simulink model "Project_Model_simulink_version_7_7_2023"  (R2021a)
settings: Solver=FixedStepDiscrete  StartTime=0.0  StopTime=10  FixedStep=0.2  RelTol=1e-3
undefined symbols (not defined in the file or in its folder): sigbuilder_block
(part 1 of 2)
settings Model: Creator=A  LastModifiedBy=91855
settings SolverCC: AlgebraicLoopSolver=TrustRegion

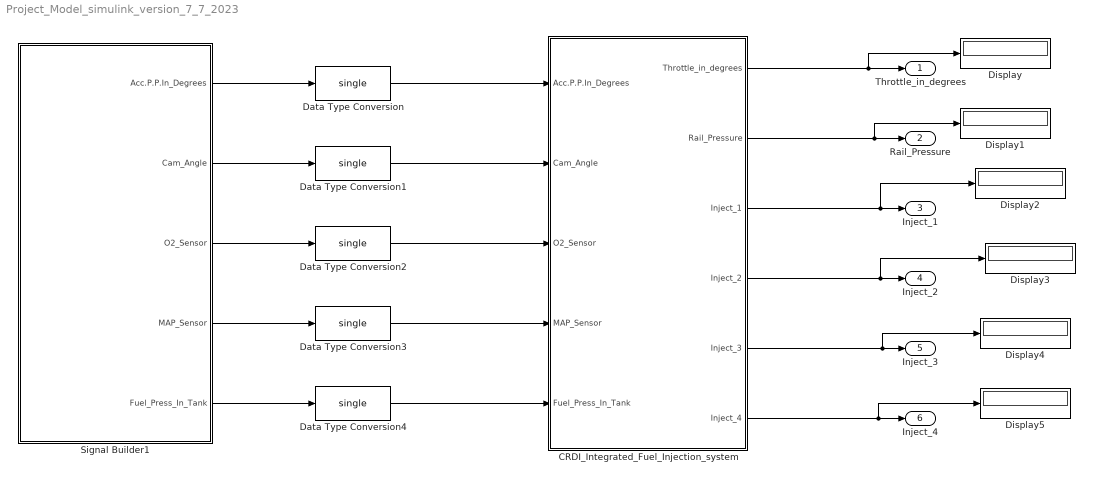
== system Project_Model_simulink_version_7_7_2023 ==
  CRDI_Integrated_Fuel_Injection_system : Subsystem
  Data Type Conversion{,1..4} (5 alike) : DataTypeConversion  OutDataTypeStr=single
  Display{,1..5} (6 alike) : Display
  Signal Builder1 : Subsystem  Tag=STV Subsys  LoadFcn=sigbuilder_block('load');  StartFcn=sigbuilder_block('start');  StopFcn=sigbuilder_block('stop');  ClipboardFcn=sigbuilder_block('clipboard');  mask(Sigbuilder block){tuvar=[0:10]}
      mask help: Simulink:masks:SigbuilderBlock_MD
      mask init:
      | if ~strcmp(get_param(bdroot(gcbh),'SimulationStatus'),'stopped') tuvar = sigbuilder_block('maskInit'); end
      settings: CopyFcn=sigbuilder_block('copy');  DeleteFcn=sigbuilder_block('delete');  ModelCloseFcn=sigbuilder_block('modelClose');  PreSaveFcn=sigbuilder_block('preSave');  PauseFcn=sigbuilder_block('pause');  ContinueFcn=sigbuilder_block('continue');  NameChangeFcn=sigbuilder_block('namechange');  OpenFcn=sigbuilder_block('open',[215 94 550.5 362.5 ]);  CloseFcn=sigbuilder_block('close');
      mask Display: plot(0, 0, 100, 100,[2, 2, 32, 32, 2], [68, 8, 8, 68, 68],[32, 2], [38, 38], [32, 19, 2],[53, 60, 44], [32, 17, 17, 2],[16, 16, 31, 31]);txt = getActiveGroup(gcbh);text(2, 100, txt,'verticalAlignment', 'top');
  Throttle_in_degrees : Outport  OutDataTypeStr=single
  Rail_Pressure : Outport  Port=2  OutDataTypeStr=single
  Inject_1 : Outport  Port=3  OutDataTypeStr=single
  Inject_2 : Outport  Port=4  OutDataTypeStr=single
  Inject_3 : Outport  Port=5  OutDataTypeStr=single
  Inject_4 : Outport  Port=6  OutDataTypeStr=single
  wires:
  CRDI_Integrated_Fuel_Injection_system/1(Throttle_in_degrees) -> Display/1, Throttle_in_degrees/1
  CRDI_Integrated_Fuel_Injection_system/2(Rail_Pressure) -> Display1/1, Rail_Pressure/1
  CRDI_Integrated_Fuel_Injection_system/3(Inject_1) -> Display2/1, Inject_1/1
  CRDI_Integrated_Fuel_Injection_system/4(Inject_2) -> Display3/1, Inject_2/1
  CRDI_Integrated_Fuel_Injection_system/5(Inject_3) -> Display4/1, Inject_3/1
  CRDI_Integrated_Fuel_Injection_system/6(Inject_4) -> Display5/1, Inject_4/1
  Data Type Conversion/1 -> CRDI_Integrated_Fuel_Injection_system/1(Acc.P.P.In_Degrees)
  Signal Builder1/2(Cam_Angle) -> Data Type Conversion1/1
  Signal Builder1/3(O2_Sensor) -> Data Type Conversion2/1
  Signal Builder1/4(MAP_Sensor) -> Data Type Conversion3/1
  Signal Builder1/5(Fuel_Press_In_Tank) -> Data Type Conversion4/1
  Data Type Conversion1/1 -> CRDI_Integrated_Fuel_Injection_system/2(Cam_Angle)
  Data Type Conversion2/1 -> CRDI_Integrated_Fuel_Injection_system/3(O2_Sensor)
  Data Type Conversion3/1 -> CRDI_Integrated_Fuel_Injection_system/4(MAP_Sensor)
  Data Type Conversion4/1 -> CRDI_Integrated_Fuel_Injection_system/5(Fuel_Press_In_Tank)
  Signal Builder1/1(Acc.P.P.In_Degrees) -> Data Type Conversion/1

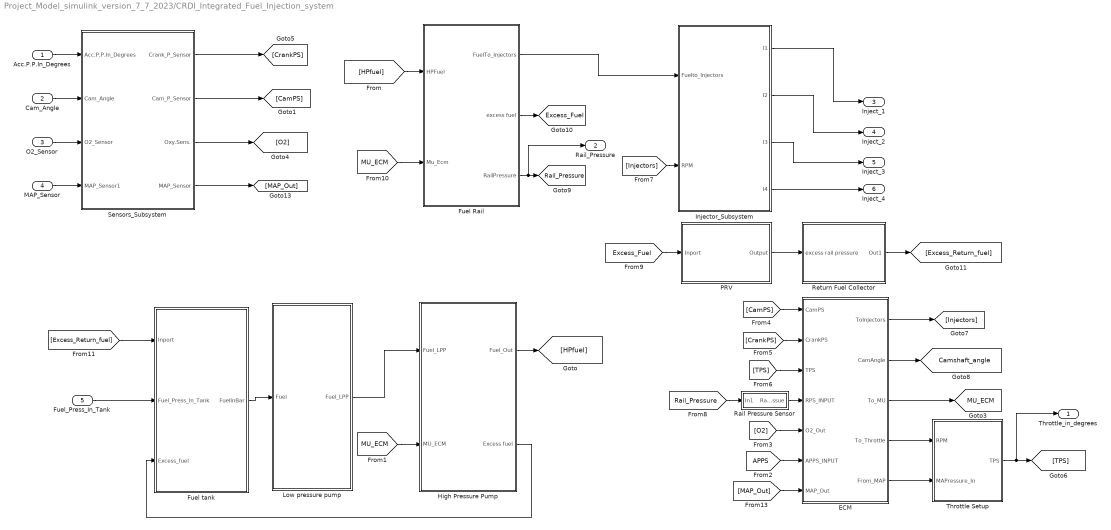
== system Project_Model_simulink_version_7_7_2023/CRDI_Integrated_Fuel_Injection_system ==
  Acc.P.P.In_Degrees : Inport  OutDataTypeStr=single
  Cam_Angle : Inport  Port=2  OutDataTypeStr=single
  O2_Sensor : Inport  Port=3  OutDataTypeStr=single
  MAP_Sensor : Inport  Port=4  OutDataTypeStr=single
  Fuel_Press_In_Tank : Inport  Port=5  OutDataTypeStr=single
  ECM : Subsystem
  Fuel Rail : Subsystem
  Fuel tank : Subsystem
  High Pressure Pump : Subsystem
  Injector_Subsystem : Subsystem
  Low pressure pump : Subsystem
  PRV : Subsystem
  Rail Pressure Sensor : Subsystem
  Return Fuel Collector : Subsystem
  Sensors_Subsystem : Subsystem
  Throttle Setup : Subsystem
  Throttle_in_degrees : Outport
  Rail_Pressure : Outport  Port=2
  Inject_1 : Outport  Port=3
  Inject_2 : Outport  Port=4
  Inject_3 : Outport  Port=5
  Inject_4 : Outport  Port=6
  tag scope: Camshaft_angle=global, Excess_Fuel=global, MU_ECM=global, Rail_Pressure=global
  wires:
  [MAP_Out] -> ECM/7(MAP_Out)
  [HPfuel] -> Fuel Rail/1(HPFuel)
  [Excess_Fuel] -> PRV/1(Inport)
  [Injectors] -> Injector_Subsystem/2(RPM)
  Throttle Setup/1(TPS) -> Throttle_in_degrees/1, [TPS]
  [O2] -> ECM/5(O2_Out)
  [MU_ECM] -> High Pressure Pump/2(MU_ECM)
  [Excess_Return_fuel] -> Fuel tank/1(Inport)
  [CamPS] -> ECM/1(CamPS)
  Rail Pressure Sensor/1(Rail Pressue) -> ECM/4(RPS_INPUT)
  [TPS] -> ECM/3(TPS)
  Fuel Rail/1(FuelTo_Injectors) -> Injector_Subsystem/1(Fuelto_Injectors)
  High Pressure Pump/2(Excess fuel) -> Fuel tank/3(Excess_fuel)
  [CrankPS] -> ECM/2(CrankPS)
  Fuel tank/1(FuelInBar) -> Low pressure pump/1(Fuel)
  Low pressure pump/1(Fuel_LPP) -> High Pressure Pump/1(Fuel_LPP)
  ECM/4(To_Throttle) -> Throttle Setup/1(RPM)
  ECM/1(ToInjectors) -> [Injectors]
  Return Fuel Collector/1(Out1) -> [Excess_Return_fuel]
  ECM/2(CamAngle) -> [Camshaft_angle]
  Fuel Rail/3(RailPressure) -> Rail_Pressure/1, [Rail_Pressure]
  High Pressure Pump/1(Fuel_Out) -> [HPfuel]
  ECM/3(To_MU) -> [MU_ECM]
  [Rail_Pressure] -> Rail Pressure Sensor/1(In1)
  Sensors_Subsystem/3(Oxy.Sens.) -> [O2]
  Sensors_Subsystem/2(Cam_P_Sensor) -> [CamPS]
  Fuel Rail/2(excess fuel) -> [Excess_Fuel]
  ECM/5(From_MAP) -> Throttle Setup/2(MAPressure_In)
  [APPS] -> ECM/6(APPS_INPUT)
  Sensors_Subsystem/1(Crank_P_Sensor) -> [CrankPS]
  Sensors_Subsystem/4(MAP_Sensor) -> [MAP_Out]
  PRV/1(Output) -> Return Fuel Collector/1(excess rail pressure)
  Injector_Subsystem/1(I1) -> Inject_1/1
  Injector_Subsystem/2(I2) -> Inject_2/1
  Injector_Subsystem/3(I3) -> Inject_3/1
  Injector_Subsystem/4(I4) -> Inject_4/1
  Fuel_Press_In_Tank/1 -> Fuel tank/2(Fuel_Press_In_Tank)
  O2_Sensor/1 -> Sensors_Subsystem/3(O2_Sensor)
  Cam_Angle/1 -> Sensors_Subsystem/2(Cam_Angle)
  MAP_Sensor/1 -> Sensors_Subsystem/4(MAP_Sensor1)
  Acc.P.P.In_Degrees/1 -> Sensors_Subsystem/1(Acc.P.P.In_Degrees)
  [MU_ECM] -> Fuel Rail/2(Mu_Ecm)

== system Project_Model_simulink_version_7_7_2023/Signal Builder1 ==
  Demux : Demux  Tag=STV Demux  Outputs=5
      settings: DisplayOption=none
  FromWs : FromWorkspace  Tag=STV FromWs  VariableName=tuvar
      SigBuilderData=|
      | common.afterFinalStr = 'Extrapolate'
      | common.sampleTime = 0
      | dataSet.timeRange = [0 4]
      | dataSet.name = 'Sheet2'
      | sbobj.Groups.Name = 'Sheet2'
      | sbobj.Groups.Signals(1).Name = 'Acc.P.P.In_Degrees'
      | sbobj.Groups.Signals(1).XData = [0 0.2 0.4 0.6 0.8 1 1.2 1.4 1.6 1.8 2 2.2 2.4 2.6 2.8 3 3.2 3.4 3.6 3.8 4]
      | sbobj.Groups.Signals(1).YData = [0 10 12 14 16 18 20 22 24 26 28 30 52 56 60 66 70 78 82 86 90]
      | sbobj.Groups.Signals(2).Name = 'Cam_Angle'
      | sbobj.Groups.Signals(2).XData = [0 0.2 0.4 0.6 0.8 1 1.2 1.4 1.6 1.8 2 2.2 2.4 2.6 2.8 3 3.2 3.4 3.6 3.8 4]
      | sbobj.Groups.Signals(2).YData = [177.5 179 180 183 184.5 222 224 225 229 267 269 270 272 274.5 313 314 315 319.2 340 345 350]
      | sbobj.Groups.Signals(3).Name = 'O2_Sensor'
      | sbobj.Groups.Signals(3).XData = [0 0.2 0.4 0.6 0.8 1 1.2 1.4 1.6 1.8 2 2.2 2.4 2.6 2.8 3 3.2 3.4 3.6 3.8 4]
      | sbobj.Groups.Signals(3).YData = [0.6 0.65 0.85 0.45 0.46 0.65 0.34 0.36 0.55 0.65 0.64 0.67 0.78 0.54 0.44 0.6 0.73 0.3 0.25 0.2 0.26]
      | sbobj.Groups.Signals(4).Name = 'MAP_Sensor'
      | sbobj.Groups.Signals(4).XData = [0 0.2 0.4 0.6 0.8 1 1.2 1.4 1.6 1.8 2 2.2 2.4 2.6 2.8 3 3.2 3.4 3.6 3.8 4]
      | sbobj.Groups.Signals(4).YData = [24 24.15 24.3 24.45 24.5 24.75 24.9 25.05 25.2 25.35 25.5 25.5 27.3 27.6 27.9 28.1 28.65 29.25 29.55 29.85 30]
      | sbobj.Groups.Signals(5).Name = 'Fuel_Press_In_Tank'
      | sbobj.Groups.Signals(5).XData = [0 0.2 0.4 0.6 0.8 1 1.2 1.4 1.6 1.8 2 2.2 2.4 2.6 2.8 3 3.2 3.4 3.6 3.8 4]
      | sbobj.Groups.Signals(5).YData = [1 1 1 1 1 1 1 1 1 1 1 1 1 1 1 1 1 1 1 1 1]
  Acc.P.P.In_Degrees : Outport  Tag=STV Outport
  Cam_Angle : Outport  Tag=STV Outport  Port=2
  O2_Sensor : Outport  Tag=STV Outport  Port=3
  MAP_Sensor : Outport  Tag=STV Outport  Port=4
  Fuel_Press_In_Tank : Outport  Tag=STV Outport  Port=5
  wires:
  Demux/1 -> Acc.P.P.In_Degrees/1
  FromWs/1 -> Demux/1
  Demux/2 -> Cam_Angle/1
  Demux/3 -> O2_Sensor/1
  Demux/4 -> MAP_Sensor/1
  Demux/5 -> Fuel_Press_In_Tank/1

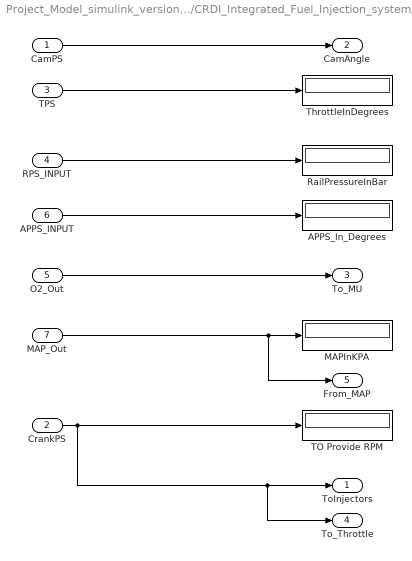
== system Project_Model_simulink_version_7_7_2023/CRDI_Integrated_Fuel_Injection_system/ECM ==
  CamPS : Inport  OutDataTypeStr=single
  CrankPS : Inport  Port=2
  TPS : Inport  Port=3
  RPS_INPUT : Inport  Port=4
  O2_Out : Inport  Port=5
  APPS_INPUT : Inport  Port=6
  MAP_Out : Inport  Port=7
  APPS_In_Degrees : Display
  MAPInKPA : Display
  RailPressureInBar : Display
  TO Provide RPM : Display
  ThrottleInDegrees : Display
  ToInjectors : Outport
  CamAngle : Outport  Port=2
  To_MU : Outport  Port=3
  To_Throttle : Outport  Port=4
  From_MAP : Outport  Port=5
  wires:
  CamPS/1 -> CamAngle/1
  APPS_INPUT/1 -> APPS_In_Degrees/1
  MAP_Out/1 -> From_MAP/1, MAPInKPA/1
  TPS/1 -> ThrottleInDegrees/1
  RPS_INPUT/1 -> RailPressureInBar/1
  CrankPS/1 -> To_Throttle/1, ToInjectors/1, TO Provide RPM/1
  O2_Out/1 -> To_MU/1

== system Project_Model_simulink_version_7_7_2023/CRDI_Integrated_Fuel_Injection_system/Fuel Rail ==
  HPFuel : Inport
  Mu_Ecm : Inport  Port=2
  1-D Lookup Table : Lookup_n-D  NumberOfTableDimensions=1  BreakpointsForDimension1=|  Table=|  InternalRulePriority=Speed  RndMeth=Simplest  InputSameDT=on
      BreakpointsForDimension1=|
      | [600
      | 730
      | 860
      | 990
      | 1120
      | 1250
      | 1380
      | 1510
      | 1640
      | 1770
      | 1900
      | 2030
      | 2160
      | 2290
      | 2420
      | 2550
      | 2680
      | 2810
      | 2940
      | 3070
      | 3200
      | 3330
      | 3460
      | 3590
      | 3720
      | 3850
      | 3980
      | 4110
      | 4240
      | 4370
      | 4500
      | 4630
      | 4760
      | 4890
      | 5020
      | 5150
      | 5280
      | 5410
      | 5540
      | 5670
      | 5800
      | 6000]
      Table=|
      | [300
      | 332
      | 364
      | 396
      | 428
      | 460
      | 492
      | 524
      | 556
      | 588
      | 620
      | 652
      | 684
      | 716
      | 748
      | 780
      | 812
      | 844
      | 876
      | 908
      | 940
      | 972
      | 1004
      | 1036
      | 1068
      | 1100
      | 1132
      | 1164
      | 1196
      | 1228
      | 1260
      | 1292
      | 1324
      | 1356
      | 1388
      | 1420
      | 1452
      | 1484
      | 1516
      | 1548
      | 1580
      | 1600]
  Product : Product
  Product1 : Product
  Subtract : Sum  Inputs=-+
  Subtract1 : Sum  Inputs=-+
  FuelTo_Injectors : Outport
  excess fuel : Outport  Port=2
  RailPressure : Outport  Port=3
  wires:
  1-D Lookup Table/1 -> Product/1, Subtract/1
  [RPM] -> 1-D Lookup Table/1
  HPFuel/1 -> Subtract1/2, Subtract/2
  Subtract/1 -> Subtract1/1, excess fuel/1
  Subtract1/1 -> Product1/1
  Product/1 -> RailPressure/1
  Product1/1 -> FuelTo_Injectors/1
  Mu_Ecm/1 -> Product1/2, Product/2

== system Project_Model_simulink_version_7_7_2023/CRDI_Integrated_Fuel_Injection_system/Fuel tank ==
  Inport : Inport
  Fuel_Press_In_Tank : Inport  Port=2
  Excess_fuel : Inport  Port=3
  ExcessFuelInBar : Display
  ExcessFuelInBar1 : Display
  FuelInBar : Outport
  wires:
  Inport/1 -> ExcessFuelInBar1/1
  Excess_fuel/1 -> ExcessFuelInBar/1
  Fuel_Press_In_Tank/1 -> FuelInBar/1

== system Project_Model_simulink_version_7_7_2023/CRDI_Integrated_Fuel_Injection_system/High Pressure Pump ==
  note: rpm=3000
      | rail pressure 902 bar
      | output = 1000 bar
      | difference = 98 bar excess
  Fuel_LPP : Inport
  MU_ECM : Inport  Port=2
  Display : Display
  Gain : Gain  Gain=160
  Metering Unit : Subsystem
  Product : Product
  Subtract : Sum  Inputs=+-
  Fuel_Out : Outport
  Excess fuel : Outport  Port=2
  wires:
  Fuel_LPP/1 -> Gain/1, Display/1
  MU_ECM/1 -> Metering Unit/1(MU_ECM)
  Metering Unit/1(Output) -> Product/2
  Gain/1 -> Subtract/1, Product/1
  Product/1 -> Subtract/2, Fuel_Out/1
  Subtract/1 -> Excess fuel/1

== system Project_Model_simulink_version_7_7_2023/CRDI_Integrated_Fuel_Injection_system/Injector_Subsystem ==
  Fuelto_Injectors : Inport
  RPM : Inport  Port=2
  Injector1 : Subsystem
  Injector2 : Subsystem
  Injector3 : Subsystem
  Injector4 : Subsystem
  I1 : Outport
  I2 : Outport  Port=2
  I3 : Outport  Port=3
  I4 : Outport  Port=4
  wires:
  RPM/1 -> Injector1/1(RPM), Injector2/1(RPM), Injector4/1(RPM), Injector3/1(RPM)
  Fuelto_Injectors/1 -> Injector1/2(HPfuel), Injector2/2(HPfuel), Injector4/2(HPfuel1), Injector3/2(HPfuel)
  Injector1/1(I1) -> I1/1
  Injector3/1(I3) -> I3/1
  Injector4/1(I4) -> I4/1
  Injector2/1(I2) -> I2/1

== system Project_Model_simulink_version_7_7_2023/CRDI_Integrated_Fuel_Injection_system/Low pressure pump ==
  Fuel : Inport
  Gain : Gain  Gain=10
  Fuel_LPP : Outport
  wires:
  Fuel/1 -> Gain/1
  Gain/1 -> Fuel_LPP/1

== system Project_Model_simulink_version_7_7_2023/CRDI_Integrated_Fuel_Injection_system/PRV ==
  Inport : Inport
  Output : Outport
  wires:
  Inport/1 -> Output/1

== system Project_Model_simulink_version_7_7_2023/CRDI_Integrated_Fuel_Injection_system/Rail Pressure Sensor ==
  In1 : Inport
  Rail Pressue : Outport
  wires:
  In1/1 -> Rail Pressue/1

== system Project_Model_simulink_version_7_7_2023/CRDI_Integrated_Fuel_Injection_system/Return Fuel Collector ==
  excess rail pressure : Inport
  Display : Display
  Out1 : Outport
  wires:
  excess rail pressure/1 -> Out1/1, Display/1

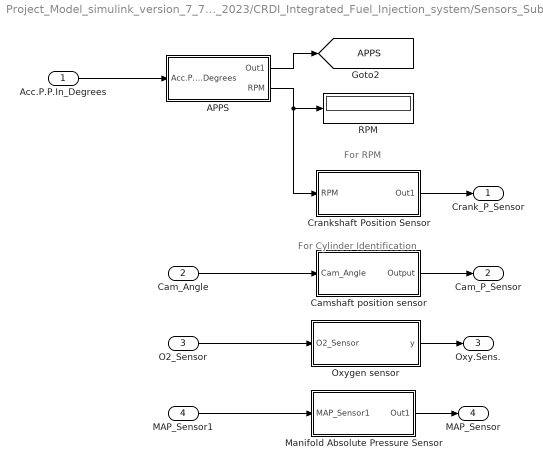
== system Project_Model_simulink_version_7_7_2023/CRDI_Integrated_Fuel_Injection_system/Sensors_Subsystem ==
  note: For Cylinder Identification
  note: For RPM
  Acc.P.P.In_Degrees : Inport  OutDataTypeStr=single
  Cam_Angle : Inport  Port=2  OutDataTypeStr=single
  O2_Sensor : Inport  Port=3  OutDataTypeStr=single
  MAP_Sensor1 : Inport  Port=4  OutDataTypeStr=single
  APPS : Subsystem
  Camshaft position sensor : Subsystem
  Crankshaft Position Sensor : Subsystem
  Manifold Absolute Pressure Sensor : Subsystem
  Oxygen sensor : Subsystem
  RPM : Display
  Crank_P_Sensor : Outport
  Cam_P_Sensor : Outport  Port=2
  Oxy.Sens. : Outport  Port=3
  MAP_Sensor : Outport  Port=4
  tag scope: APPS=global
  wires:
  Oxygen sensor/1(y) -> Oxy.Sens./1
  APPS/2(RPM) -> Crankshaft Position Sensor/1(RPM), RPM/1
  Camshaft position sensor/1(Output) -> Cam_P_Sensor/1
  Crankshaft Position Sensor/1(Out1) -> Crank_P_Sensor/1
  APPS/1(Out1) -> [APPS]
  Manifold Absolute Pressure Sensor/1(Out1) -> MAP_Sensor/1
  Acc.P.P.In_Degrees/1 -> APPS/1(Acc.P.P.In_Degrees)
  Cam_Angle/1 -> Camshaft position sensor/1(Cam_Angle)
  O2_Sensor/1 -> Oxygen sensor/1(O2_Sensor)
  MAP_Sensor1/1 -> Manifold Absolute Pressure Sensor/1(MAP_Sensor1)

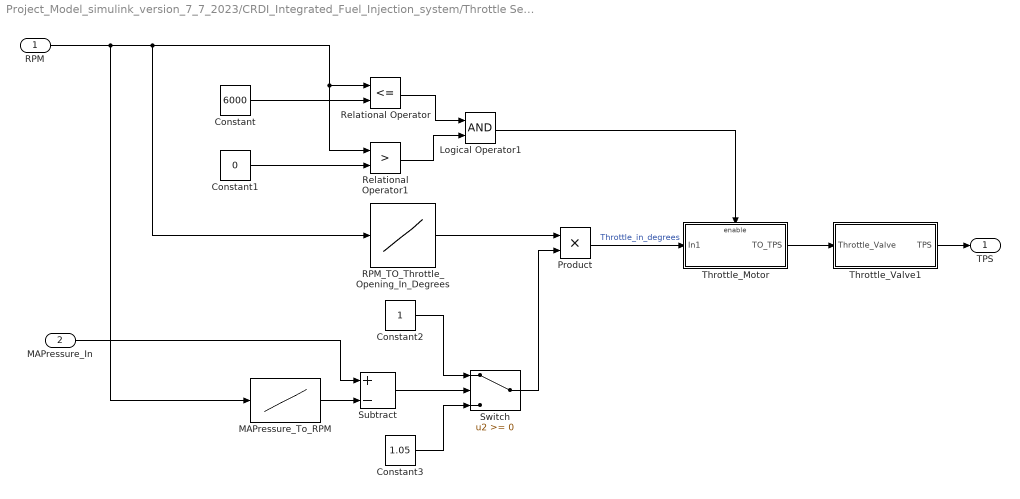
== system Project_Model_simulink_version_7_7_2023/CRDI_Integrated_Fuel_Injection_system/Throttle Setup ==
  RPM : Inport
  MAPressure_In : Inport  Port=2
  Constant : Constant  Value=6000
  Constant1 : Constant  Value=0
  Constant2 : Constant
  Constant3 : Constant  Value=1.05
  Logical Operator1 : Logic  AllPortsSameDT=off  OutDataTypeStr=boolean
  MAPressure_To_RPM : Lookup_n-D  NumberOfTableDimensions=1  BreakpointsForDimension1=|  Table=|  InternalRulePriority=Speed  RndMeth=Simplest  InputSameDT=on
      BreakpointsForDimension1=|
      | [600
      | 730
      | 860
      | 990
      | 1120
      | 1250
      | 1380
      | 1510
      | 1640
      | 1770
      | 1900
      | 2030
      | 2160
      | 2290
      | 2420
      | 2550
      | 2680
      | 2810
      | 2940
      | 3070
      | 3200
      | 3330
      | 3460
      | 3590
      | 3720
      | 3850
      | 3980
      | 4110
      | 4240
      | 4370
      | 4500
      | 4630
      | 4760
      | 4890
      | 5020
      | 5150
      | 5280
      | 5410
      | 5540
      | 5670
      | 5800
      | 6000]
      Table=|
      | [24
      | 24.2
      | 24.3
      | 24.5
      | 24.6
      | 24.8
      | 24.9
      | 25.1
      | 25.2
      | 25.4
      | 25.5
      | 25.7
      | 25.8
      | 26.0
      | 26.1
      | 26.3
      | 26.4
      | 26.6
      | 26.7
      | 26.9
      | 27.0
      | 27.2
      | 27.3
      | 27.5
      | 27.6
      | 27.8
      | 27.9
      | 28.1
      | 28.2
      | 28.4
      | 28.5
      | 28.7
      | 28.8
      | 29.0
      | 29.1
      | 29.3
      | 29.4
      | 29.5
      | 29.7
      | 29.8
      | 29.9
      | 30]
  Product : Product
  RPM_TO_Throttle_Opening_In_Degrees : Lookup_n-D  NumberOfTableDimensions=1  BreakpointsForDimension1=|  Table=|  InternalRulePriority=Speed  RndMeth=Simplest  InputSameDT=on
      BreakpointsForDimension1=|
      | [600
      | 730
      | 860
      | 990
      | 1120
      | 1250
      | 1380
      | 1510
      | 1640
      | 1770
      | 1900
      | 2030
      | 2160
      | 2290
      | 2420
      | 2550
      | 2680
      | 2810
      | 2940
      | 3070
      | 3200
      | 3330
      | 3460
      | 3590
      | 3720
      | 3850
      | 3980
      | 4110
      | 4240
      | 4370
      | 4500
      | 4630
      | 4760
      | 4890
      | 5020
      | 5150
      | 5280
      | 5410
      | 5540
      | 5670
      | 5800
      | 6000]
      Table=|
      | [8
      | 10
      | 12
      | 14
      | 16
      | 18
      | 20
      | 22
      | 24
      | 26
      | 28
      | 30
      | 32
      | 34
      | 36
      | 38
      | 40
      | 42
      | 44
      | 46
      | 48
      | 50
      | 52
      | 54
      | 56
      | 58
      | 60
      | 62
      | 64
      | 66
      | 68
      | 70
      | 72
      | 74
      | 76
      | 78
      | 80
      | 82
      | 84
      | 86
      | 88
      | 90]
  Relational Operator : RelationalOperator  Operator=<=  OutDataTypeStr=boolean  RndMeth=Simplest
  Relational Operator1 : RelationalOperator  Operator=>  OutDataTypeStr=boolean  RndMeth=Simplest
  Subtract : Sum  Inputs=+-
  Switch : Switch
  Throttle_Motor : Subsystem  TreatAsAtomicUnit=on
  Throttle_Valve1 : Subsystem
  TPS : Outport
  wires:
  Throttle_Motor/1(TO_TPS) -> Throttle_Valve1/1(Throttle_Valve)
  Constant/1 -> Relational Operator/2
  Subtract/1 -> Switch/2
  MAPressure_To_RPM/1 -> Subtract/2
  Constant2/1 -> Switch/1
  Relational Operator/1 -> Logical Operator1/1
  Constant3/1 -> Switch/3
  Relational Operator1/1 -> Logical Operator1/2
  Switch/1 -> Product/2
  MAPressure_In/1 -> Subtract/1
  Logical Operator1/1 -> Throttle_Motor/Enable
  Product/1 -> Throttle_Motor/1(In1)  "Throttle_in_degrees"
  RPM/1 -> MAPressure_To_RPM/1, RPM_TO_Throttle_Opening_In_Degrees/1, Relational Operator1/1, Relational Operator/1
  Constant1/1 -> Relational Operator1/2
  RPM_TO_Throttle_Opening_In_Degrees/1 -> Product/1
  Throttle_Valve1/1(TPS) -> TPS/1

== system Project_Model_simulink_version_7_7_2023/CRDI_Integrated_Fuel_Injection_system/High Pressure Pump/Metering Unit ==
  note: if fuel pressure in rail is as per the required in specific rpm then duty cycle is 15 % if pressure is more duty cylce will increase to 20 % until pressure in rail is as per required
  MU_ECM : Inport
  Output : Outport
  wires:
  MU_ECM/1 -> Output/1

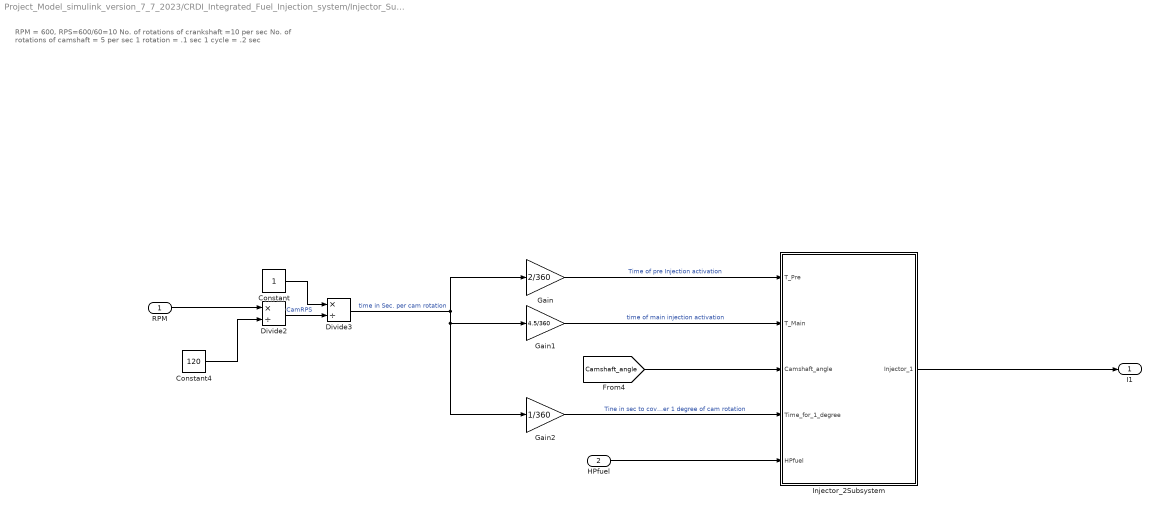
== system Project_Model_simulink_version_7_7_2023/CRDI_Integrated_Fuel_Injection_system/Injector_Subsystem/Injector1 ==
  note: RPM = 600,
      | RPS=600/60=10
      | No. of rotations of crankshaft =10 per sec
      | No. of rotations of camshaft = 5 per sec
      | 1 rotation = .1 sec
      | 1 cycle = .2 sec
  RPM : Inport
  HPfuel : Inport  Port=2
  Constant : Constant  OutDataTypeStr=single
  Constant4 : Constant  Value=120
  Divide2 : Product  Inputs=*/  OutDataTypeStr=single
  Divide3 : Product  Inputs=*/  OutDataTypeStr=single
  Gain : Gain  Gain=2/360
  Gain1 : Gain  Gain=4.5/360
  Gain2 : Gain  Gain=1/360
  Injector_2Subsystem : Subsystem  TreatAsAtomicUnit=on
  I1 : Outport
  wires:
  Gain2/1 -> Injector_2Subsystem/4(Time_for_1_degree)  "Tine in sec to cover 1 degree of cam rotation"
  Gain/1 -> Injector_2Subsystem/1(T_Pre)  "Time of pre Injection activation"
  RPM/1 -> Divide2/1
  Divide3/1 -> Gain/1, Gain2/1, Gain1/1  "time in Sec. per cam rotation"
  Injector_2Subsystem/1(Injector_1) -> I1/1
  Divide2/1 -> Divide3/2  "CamRPS"
  [Camshaft_angle] -> Injector_2Subsystem/3(Camshaft_angle)
  HPfuel/1 -> Injector_2Subsystem/5(HPfuel)
  Gain1/1 -> Injector_2Subsystem/2(T_Main)  "time of main injection activation"
  Constant/1 -> Divide3/1
  Constant4/1 -> Divide2/2

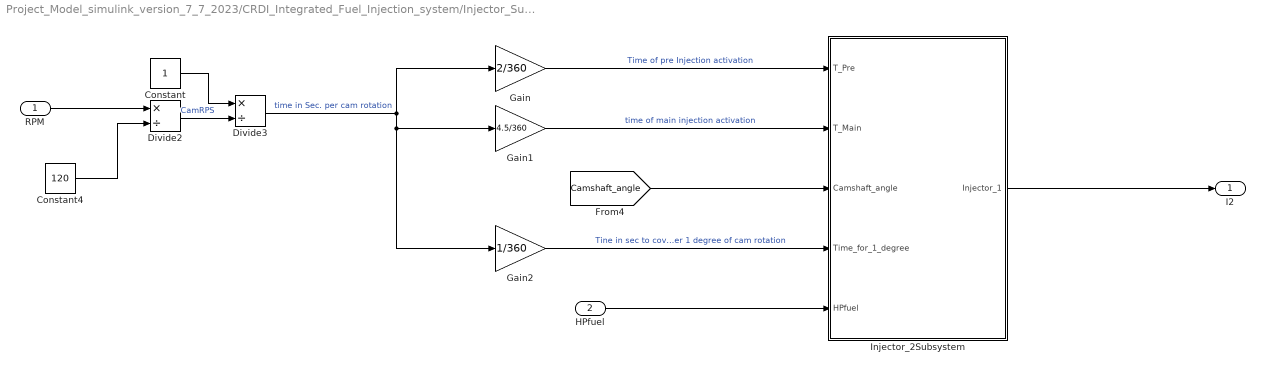
== system Project_Model_simulink_version_7_7_2023/CRDI_Integrated_Fuel_Injection_system/Injector_Subsystem/Injector2 ==
  RPM : Inport
  HPfuel : Inport  Port=2
  Constant : Constant  OutDataTypeStr=single
  Constant4 : Constant  Value=120
  Divide2 : Product  Inputs=*/  OutDataTypeStr=single
  Divide3 : Product  Inputs=*/  OutDataTypeStr=single
  Gain : Gain  Gain=2/360
  Gain1 : Gain  Gain=4.5/360
  Gain2 : Gain  Gain=1/360
  Injector_2Subsystem : Subsystem  TreatAsAtomicUnit=on
  I2 : Outport
  wires:
  Gain2/1 -> Injector_2Subsystem/4(Time_for_1_degree)  "Tine in sec to cover 1 degree of cam rotation"
  Gain/1 -> Injector_2Subsystem/1(T_Pre)  "Time of pre Injection activation"
  RPM/1 -> Divide2/1
  Divide3/1 -> Gain/1, Gain2/1, Gain1/1  "time in Sec. per cam rotation"
  Injector_2Subsystem/1(Injector_1) -> I2/1
  Divide2/1 -> Divide3/2  "CamRPS"
  [Camshaft_angle] -> Injector_2Subsystem/3(Camshaft_angle)
  HPfuel/1 -> Injector_2Subsystem/5(HPfuel)
  Gain1/1 -> Injector_2Subsystem/2(T_Main)  "time of main injection activation"
  Constant/1 -> Divide3/1
  Constant4/1 -> Divide2/2

== system Project_Model_simulink_version_7_7_2023/CRDI_Integrated_Fuel_Injection_system/Injector_Subsystem/Injector3 ==
  RPM : Inport
  HPfuel : Inport  Port=2
  Constant : Constant  OutDataTypeStr=single
  Constant4 : Constant  Value=120
  Divide2 : Product  Inputs=*/  OutDataTypeStr=single
  Divide3 : Product  Inputs=*/  OutDataTypeStr=single
  Gain : Gain  Gain=2/360
  Gain1 : Gain  Gain=4.5/360
  Gain2 : Gain  Gain=1/360
  Injector_2Subsystem : Subsystem  TreatAsAtomicUnit=on
  I3 : Outport
  wires:
  Injector_2Subsystem/1(Injector_1) -> I3/1
  [Camshaft_angle] -> Injector_2Subsystem/3(Camshaft_angle)
  Gain2/1 -> Injector_2Subsystem/4(Time_for_1_degree)  "Tine in sec to cover 1 degree of cam rotation"
  HPfuel/1 -> Injector_2Subsystem/5(HPfuel)
  Divide3/1 -> Gain/1, Gain2/1, Gain1/1  "time in Sec. per cam rotation"
  Divide2/1 -> Divide3/2  "CamRPS"
  Gain/1 -> Injector_2Subsystem/1(T_Pre)  "Time of pre Injection activation"
  Constant/1 -> Divide3/1
  Constant4/1 -> Divide2/2
  RPM/1 -> Divide2/1
  Gain1/1 -> Injector_2Subsystem/2(T_Main)  "time of main injection activation"

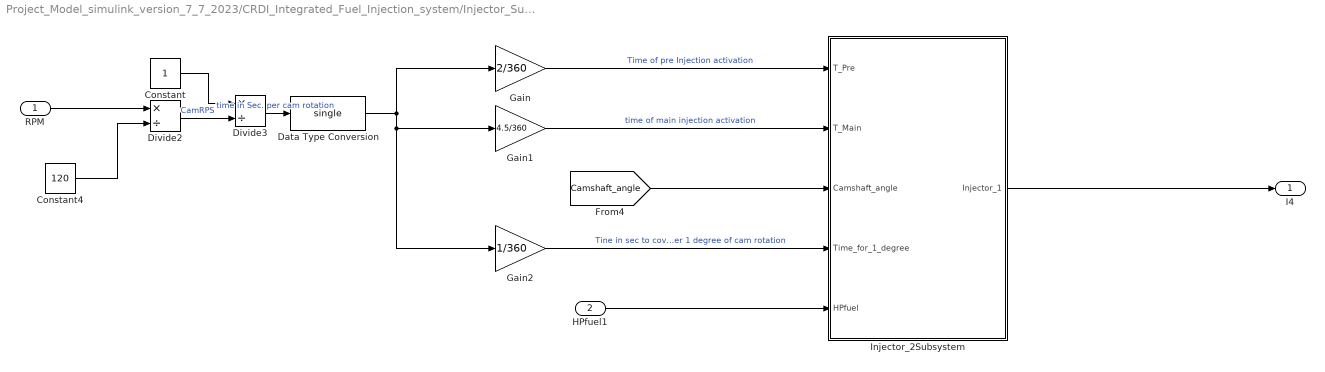
== system Project_Model_simulink_version_7_7_2023/CRDI_Integrated_Fuel_Injection_system/Injector_Subsystem/Injector4 ==
  RPM : Inport
  HPfuel1 : Inport  Port=2
  Constant : Constant
  Constant4 : Constant  Value=120
  Data Type Conversion : DataTypeConversion  OutDataTypeStr=single
  Divide2 : Product  Inputs=*/
  Divide3 : Product  Inputs=*/
  Gain : Gain  Gain=2/360
  Gain1 : Gain  Gain=4.5/360
  Gain2 : Gain  Gain=1/360
  Injector_2Subsystem : Subsystem  TreatAsAtomicUnit=on
  I4 : Outport
  wires:
  Gain2/1 -> Injector_2Subsystem/4(Time_for_1_degree)  "Tine in sec to cover 1 degree of cam rotation"
  Gain/1 -> Injector_2Subsystem/1(T_Pre)  "Time of pre Injection activation"
  RPM/1 -> Divide2/1
  Divide3/1 -> Data Type Conversion/1  "time in Sec. per cam rotation"
  Injector_2Subsystem/1(Injector_1) -> I4/1
  Divide2/1 -> Divide3/2  "CamRPS"
  [Camshaft_angle] -> Injector_2Subsystem/3(Camshaft_angle)
  HPfuel1/1 -> Injector_2Subsystem/5(HPfuel)
  Gain1/1 -> Injector_2Subsystem/2(T_Main)  "time of main injection activation"
  Constant/1 -> Divide3/1
  Constant4/1 -> Divide2/2
  Data Type Conversion/1 -> Gain/1, Gain2/1, Gain1/1

== system Project_Model_simulink_version_7_7_2023/CRDI_Integrated_Fuel_Injection_system/Sensors_Subsystem/APPS ==
  Acc.P.P.In_Degrees : Inport  OutDataTypeStr=single
  1-D Lookup Table : Lookup_n-D  NumberOfTableDimensions=1  BreakpointsForDimension1=|  BreakpointsForDimension1DataTypeStr=double  Table=|  TableDataTypeStr=double  ExtrapMethod=Clip  InternalRulePriority=Speed  RndMeth=Simplest  InputSameDT=on
      BreakpointsForDimension1=|
      | [0
      | 10
      | 12
      | 14
      | 16
      | 18
      | 20
      | 22
      | 24
      | 26
      | 28
      | 30
      | 32
      | 34
      | 36
      | 38
      | 40
      | 42
      | 44
      | 46
      | 48
      | 50
      | 52
      | 54
      | 56
      | 58
      | 60
      | 62
      | 64
      | 66
      | 68
      | 70
      | 72
      | 74
      | 76
      | 78
      | 80
      | 82
      | 84
      | 86
      | 88
      | 90]
      Table=|
      | [600
      | 730
      | 860
      | 990
      | 1120
      | 1250
      | 1380
      | 1510
      | 1640
      | 1770
      | 1900
      | 2030
      | 2160
      | 2290
      | 2420
      | 2550
      | 2680
      | 2810
      | 2940
      | 3070
      | 3200
      | 3330
      | 3460
      | 3590
      | 3720
      | 3850
      | 3980
      | 4110
      | 4240
      | 4370
      | 4500
      | 4630
      | 4760
      | 4890
      | 5020
      | 5150
      | 5280
      | 5410
      | 5540
      | 5670
      | 5800
      | 6000]
  Out1 : Outport
  RPM : Outport  Port=2
  tag scope: RPM=global
  wires:
  1-D Lookup Table/1 -> [RPM], RPM/1
  Acc.P.P.In_Degrees/1 -> 1-D Lookup Table/1, Out1/1

== system Project_Model_simulink_version_7_7_2023/CRDI_Integrated_Fuel_Injection_system/Sensors_Subsystem/Camshaft position sensor ==
  Cam_Angle : Inport  OutDataTypeStr=single
  Output : Outport  OutDataTypeStr=single
  wires:
  Cam_Angle/1 -> Output/1  "Cam_angle"

== system Project_Model_simulink_version_7_7_2023/CRDI_Integrated_Fuel_Injection_system/Sensors_Subsystem/Crankshaft Position Sensor ==
  RPM : Inport
  Out1 : Outport
  wires:
  RPM/1 -> Out1/1

== system Project_Model_simulink_version_7_7_2023/CRDI_Integrated_Fuel_Injection_system/Sensors_Subsystem/Manifold Absolute Pressure Sensor ==
  MAP_Sensor1 : Inport  OutDataTypeStr=single
  Out1 : Outport  OutDataTypeStr=single
  wires:
  MAP_Sensor1/1 -> Out1/1

== system Project_Model_simulink_version_7_7_2023/CRDI_Integrated_Fuel_Injection_system/Sensors_Subsystem/Oxygen sensor ==
  O2_Sensor : Inport  OutDataTypeStr=single
  Data Type Conversion : DataTypeConversion  OutDataTypeStr=single
  MATLAB Function : MATLAB Function  TreatAsAtomicUnit=on
  y : Outport  OutDataTypeStr=single
  wires:
  MATLAB Function/1(out) -> Data Type Conversion/1
  O2_Sensor/1 -> MATLAB Function/1(u)
  Data Type Conversion/1 -> y/1

== system Project_Model_simulink_version_7_7_2023/CRDI_Integrated_Fuel_Injection_system/Throttle Setup/Throttle_Motor ==
  In1 : Inport
  Enable : EnablePort
  Constant : Constant  Value=90
  Switch : Switch  Criteria=u2 > Threshold  Threshold=90
  TO_TPS : Outport
  wires:
  In1/1 -> Switch/3, Switch/2
  Switch/1 -> TO_TPS/1
  Constant/1 -> Switch/1

== system Project_Model_simulink_version_7_7_2023/CRDI_Integrated_Fuel_Injection_system/Throttle Setup/Throttle_Valve1 ==
  Throttle_Valve : Inport
  TPS : Outport
  wires:
  Throttle_Valve/1 -> TPS/1

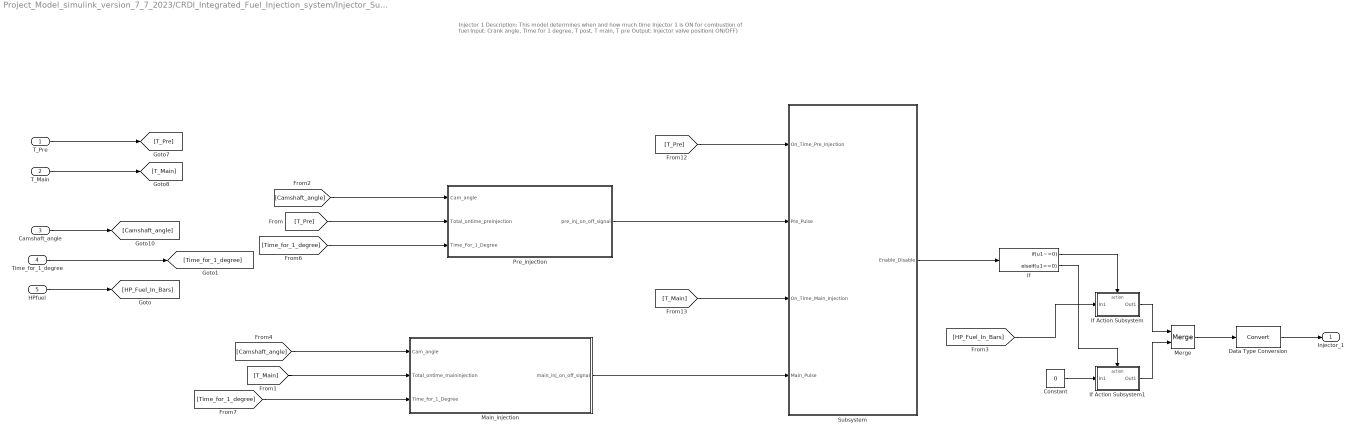
== system Project_Model_simulink_version_7_7_2023/CRDI_Integrated_Fuel_Injection_system/Injector_Subsystem/Injector1/Injector_2Subsystem ==
  note: Injector 1
      | Description: This model determines when and how much time Injector 1 is ON for combustion of fuel
      | Input: Crank angle, TIme for 1 degree, T post, T main, T pre
      | Output: Injector valve position( ON/OFF)
  T_Pre : Inport
  T_Main : Inport  Port=2
  Camshaft_angle : Inport  Port=3
  Time_for_1_degree : Inport  Port=4
  HPfuel : Inport  Port=5
  Constant : Constant  Value=0  OutDataTypeStr=single
  Data Type Conversion : DataTypeConversion
  If : If  IfExpression=u1~=0  ElseIfExpressions=u1==0  ShowElse=off
  If Action Subsystem : Subsystem  TreatAsAtomicUnit=on
  If Action Subsystem1 : Subsystem  TreatAsAtomicUnit=on
  Main_injection : Subsystem  TreatAsAtomicUnit=on
  Merge : Merge
  Pre_injection : Subsystem  TreatAsAtomicUnit=on
  Subsystem : Subsystem
  Injector_1 : Outport  OutDataTypeStr=single
  wires:
  T_Pre/1 -> [T_Pre]
  T_Main/1 -> [T_Main]
  Time_for_1_degree/1 -> [Time_for_1_degree]
  [Time_for_1_degree] -> Main_injection/3(Time_for_1_Degree)
  [T_Main] -> Main_injection/2(Total_ontime_maininjection)
  [Camshaft_angle] -> Main_injection/1(Cam_angle)
  [Time_for_1_degree] -> Pre_injection/3(Time_For_1_Degree)
  [Camshaft_angle] -> Pre_injection/1(Cam_angle)
  [T_Pre] -> Pre_injection/2(Total_ontime_preinjection)
  Subsystem/1(Enable_Disable) -> If/1
  Merge/1 -> Data Type Conversion/1
  [T_Pre] -> Subsystem/1(On_Time_Pre_Injection)
  [T_Main] -> Subsystem/3(On_Time_Main_Injection)
  Main_injection/1(main_inj_on_off_signal) -> Subsystem/4(Main_Pulse)
  Pre_injection/1(pre_inj_on_off_signal) -> Subsystem/2(Pre_Pulse)
  [HP_Fuel_In_Bars] -> If Action Subsystem/1(In1)
  HPfuel/1 -> [HP_Fuel_In_Bars]
  Camshaft_angle/1 -> [Camshaft_angle]
  If/1 -> If Action Subsystem/Action
  If Action Subsystem/1(Out1) -> Merge/1
  If/2 -> If Action Subsystem1/Action
  Constant/1 -> If Action Subsystem1/1(In1)
  If Action Subsystem1/1(Out1) -> Merge/2
  Data Type Conversion/1 -> Injector_1/1

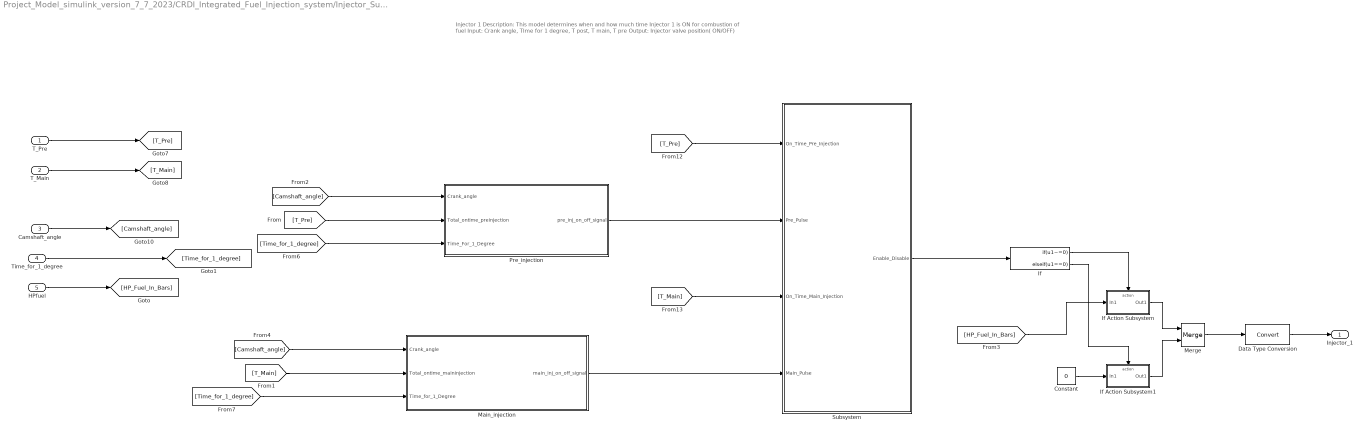
== system Project_Model_simulink_version_7_7_2023/CRDI_Integrated_Fuel_Injection_system/Injector_Subsystem/Injector2/Injector_2Subsystem ==
  note: Injector 1
      | Description: This model determines when and how much time Injector 1 is ON for combustion of fuel
      | Input: Crank angle, TIme for 1 degree, T post, T main, T pre
      | Output: Injector valve position( ON/OFF)
  T_Pre : Inport
  T_Main : Inport  Port=2
  Camshaft_angle : Inport  Port=3
  Time_for_1_degree : Inport  Port=4
  HPfuel : Inport  Port=5
  Constant : Constant  Value=0  OutDataTypeStr=single
  Data Type Conversion : DataTypeConversion
  If : If  IfExpression=u1~=0  ElseIfExpressions=u1==0  ShowElse=off
  If Action Subsystem : Subsystem  TreatAsAtomicUnit=on
  If Action Subsystem1 : Subsystem  TreatAsAtomicUnit=on
  Main_injection : Subsystem  TreatAsAtomicUnit=on
  Merge : Merge
  Pre_injection : Subsystem  TreatAsAtomicUnit=on
  Subsystem : Subsystem
  Injector_1 : Outport
  wires:
  T_Pre/1 -> [T_Pre]
  T_Main/1 -> [T_Main]
  Time_for_1_degree/1 -> [Time_for_1_degree]
  [Time_for_1_degree] -> Main_injection/3(Time_for_1_Degree)
  [T_Main] -> Main_injection/2(Total_ontime_maininjection)
  [Camshaft_angle] -> Main_injection/1(Crank_angle)
  [Time_for_1_degree] -> Pre_injection/3(Time_For_1_Degree)
  [Camshaft_angle] -> Pre_injection/1(Crank_angle)
  [T_Pre] -> Pre_injection/2(Total_ontime_preinjection)
  [T_Pre] -> Subsystem/1(On_Time_Pre_Injection)
  [T_Main] -> Subsystem/3(On_Time_Main_Injection)
  Main_injection/1(main_inj_on_off_signal) -> Subsystem/4(Main_Pulse)
  Pre_injection/1(pre_inj_on_off_signal) -> Subsystem/2(Pre_Pulse)
  HPfuel/1 -> [HP_Fuel_In_Bars]
  Camshaft_angle/1 -> [Camshaft_angle]
  Subsystem/1(Enable_Disable) -> If/1
  If/2 -> If Action Subsystem1/Action
  Data Type Conversion/1 -> Injector_1/1
  Constant/1 -> If Action Subsystem1/1(In1)
  If Action Subsystem1/1(Out1) -> Merge/2
  [HP_Fuel_In_Bars] -> If Action Subsystem/1(In1)
  If Action Subsystem/1(Out1) -> Merge/1
  If/1 -> If Action Subsystem/Action
  Merge/1 -> Data Type Conversion/1

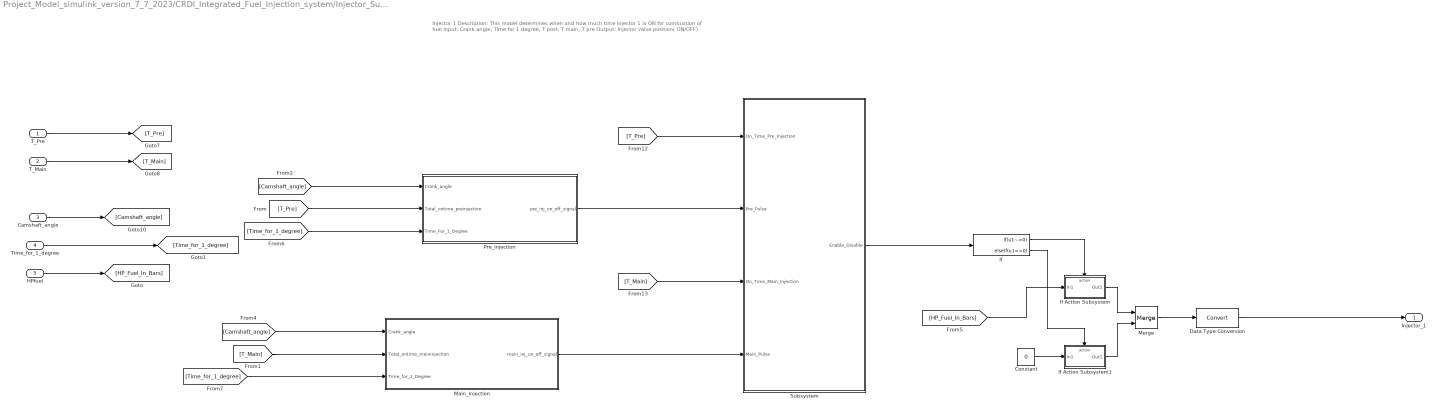
== system Project_Model_simulink_version_7_7_2023/CRDI_Integrated_Fuel_Injection_system/Injector_Subsystem/Injector3/Injector_2Subsystem ==
  note: Injector 1
      | Description: This model determines when and how much time Injector 1 is ON for combustion of fuel
      | Input: Crank angle, TIme for 1 degree, T post, T main, T pre
      | Output: Injector valve position( ON/OFF)
  T_Pre : Inport
  T_Main : Inport  Port=2
  Camshaft_angle : Inport  Port=3
  Time_for_1_degree : Inport  Port=4
  HPfuel : Inport  Port=5
  Constant : Constant  Value=0  OutDataTypeStr=single
  Data Type Conversion : DataTypeConversion
  If : If  IfExpression=u1~=0  ElseIfExpressions=u1==0  ShowElse=off
  If Action Subsystem : Subsystem  TreatAsAtomicUnit=on
  If Action Subsystem1 : Subsystem  TreatAsAtomicUnit=on
  Main_injection : Subsystem  TreatAsAtomicUnit=on
  Merge : Merge
  Pre_injection : Subsystem  TreatAsAtomicUnit=on
  Subsystem : Subsystem
  Injector_1 : Outport
  wires:
  T_Pre/1 -> [T_Pre]
  T_Main/1 -> [T_Main]
  Time_for_1_degree/1 -> [Time_for_1_degree]
  [Time_for_1_degree] -> Main_injection/3(Time_for_1_Degree)
  [T_Main] -> Main_injection/2(Total_ontime_maininjection)
  [Camshaft_angle] -> Main_injection/1(Crank_angle)
  [Time_for_1_degree] -> Pre_injection/3(Time_For_1_Degree)
  [Camshaft_angle] -> Pre_injection/1(Crank_angle)
  [T_Pre] -> Pre_injection/2(Total_ontime_preinjection)
  [T_Pre] -> Subsystem/1(On_Time_Pre_Injection)
  [T_Main] -> Subsystem/3(On_Time_Main_Injection)
  Main_injection/1(main_inj_on_off_signal) -> Subsystem/4(Main_Pulse)
  Pre_injection/1(pre_inj_on_off_signal) -> Subsystem/2(Pre_Pulse)
  HPfuel/1 -> [HP_Fuel_In_Bars]
  Camshaft_angle/1 -> [Camshaft_angle]
  Merge/1 -> Data Type Conversion/1
  [HP_Fuel_In_Bars] -> If Action Subsystem/1(In1)
  If/1 -> If Action Subsystem/Action
  If Action Subsystem/1(Out1) -> Merge/1
  Subsystem/1(Enable_Disable) -> If/1
  Constant/1 -> If Action Subsystem1/1(In1)
  Data Type Conversion/1 -> Injector_1/1
  If Action Subsystem1/1(Out1) -> Merge/2
  If/2 -> If Action Subsystem1/Action

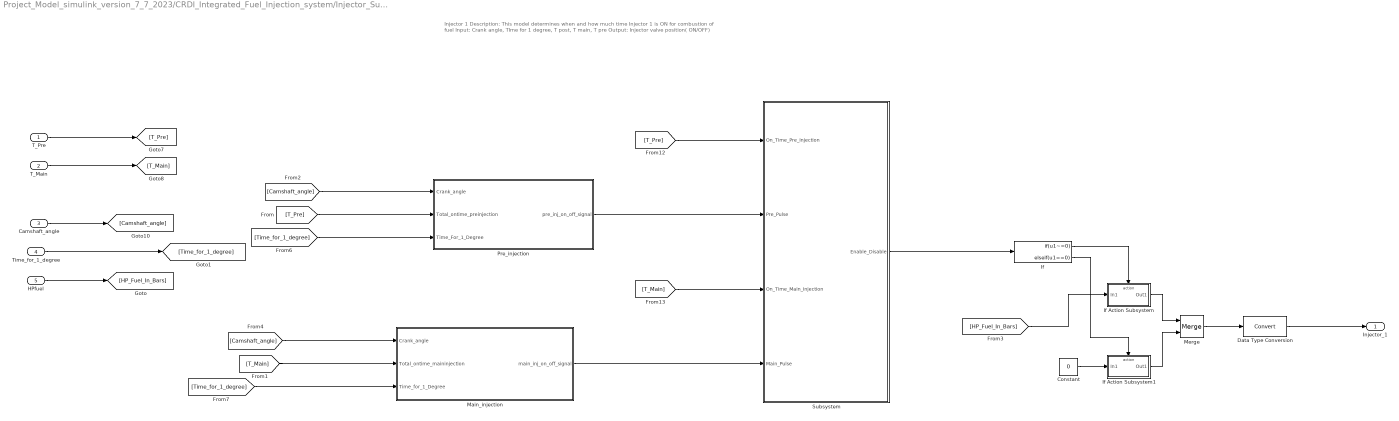
== system Project_Model_simulink_version_7_7_2023/CRDI_Integrated_Fuel_Injection_system/Injector_Subsystem/Injector4/Injector_2Subsystem ==
  note: Injector 1
      | Description: This model determines when and how much time Injector 1 is ON for combustion of fuel
      | Input: Crank angle, TIme for 1 degree, T post, T main, T pre
      | Output: Injector valve position( ON/OFF)
  T_Pre : Inport
  T_Main : Inport  Port=2
  Camshaft_angle : Inport  Port=3
  Time_for_1_degree : Inport  Port=4
  HPfuel : Inport  Port=5
  Constant : Constant  Value=0  OutDataTypeStr=single
  Data Type Conversion : DataTypeConversion
  If : If  IfExpression=u1~=0  ElseIfExpressions=u1==0  ShowElse=off
  If Action Subsystem : Subsystem  TreatAsAtomicUnit=on
  If Action Subsystem1 : Subsystem  TreatAsAtomicUnit=on
  Main_injection : Subsystem  TreatAsAtomicUnit=on
  Merge : Merge
  Pre_injection : Subsystem  TreatAsAtomicUnit=on
  Subsystem : Subsystem
  Injector_1 : Outport
  wires:
  T_Pre/1 -> [T_Pre]
  T_Main/1 -> [T_Main]
  Time_for_1_degree/1 -> [Time_for_1_degree]
  [Time_for_1_degree] -> Main_injection/3(Time_for_1_Degree)
  [T_Main] -> Main_injection/2(Total_ontime_maininjection)
  [Camshaft_angle] -> Main_injection/1(Crank_angle)
  [Time_for_1_degree] -> Pre_injection/3(Time_For_1_Degree)
  [Camshaft_angle] -> Pre_injection/1(Crank_angle)
  [T_Pre] -> Pre_injection/2(Total_ontime_preinjection)
  Subsystem/1(Enable_Disable) -> If/1
  [T_Pre] -> Subsystem/1(On_Time_Pre_Injection)
  [T_Main] -> Subsystem/3(On_Time_Main_Injection)
  Main_injection/1(main_inj_on_off_signal) -> Subsystem/4(Main_Pulse)
  Pre_injection/1(pre_inj_on_off_signal) -> Subsystem/2(Pre_Pulse)
  HPfuel/1 -> [HP_Fuel_In_Bars]
  Camshaft_angle/1 -> [Camshaft_angle]
  Merge/1 -> Data Type Conversion/1
  [HP_Fuel_In_Bars] -> If Action Subsystem/1(In1)
  If/1 -> If Action Subsystem/Action
  If Action Subsystem/1(Out1) -> Merge/1
  Constant/1 -> If Action Subsystem1/1(In1)
  Data Type Conversion/1 -> Injector_1/1
  If Action Subsystem1/1(Out1) -> Merge/2
  If/2 -> If Action Subsystem1/Action

== system Project_Model_simulink_version_7_7_2023/CRDI_Integrated_Fuel_Injection_system/Injector_Subsystem/Injector1/Injector_2Subsystem/If Action Subsystem ==
  In1 : Inport  OutDataTypeStr=single
  Action Port : ActionPort  ActionPortLabel=if(u1~=0)
  Out1 : Outport  OutDataTypeStr=single
  wires:
  In1/1 -> Out1/1

== system Project_Model_simulink_version_7_7_2023/CRDI_Integrated_Fuel_Injection_system/Injector_Subsystem/Injector1/Injector_2Subsystem/If Action Subsystem1 ==
  In1 : Inport  OutDataTypeStr=single
  Action Port : ActionPort  ActionPortLabel=elseif(u1==0)
  Out1 : Outport  OutDataTypeStr=single
  wires:
  In1/1 -> Out1/1

== system Project_Model_simulink_version_7_7_2023/CRDI_Integrated_Fuel_Injection_system/Injector_Subsystem/Injector1/Injector_2Subsystem/Main_injection ==
  Cam_angle : Inport  OutDataTypeStr=single
  Total_ontime_maininjection : Inport  Port=2  OutDataTypeStr=single
  Time_for_1_Degree : Inport  Port=3  OutDataTypeStr=single
  Add : Sum  AccumDataTypeStr=single
      settings: AttributesFormatString=AccumDataTypeStr=%<AccumDataTypeStr>
  Divide : Product  Inputs=*/  OutDataTypeStr=single
  Logical Operator : Logic  AllPortsSameDT=off  OutDataTypeStr=boolean
  Main_Inj_trg_angle_inj1 : Constant  Value=180
  Main_Inj_trg_angle_inj2 : Constant  Value=180
  Relational Operator : RelationalOperator  OutDataTypeStr=boolean  RndMeth=Simplest
  Relational Operator1 : RelationalOperator  Operator=<=  OutDataTypeStr=boolean  RndMeth=Simplest
  main_inj_on_off_signal : Outport  VectorParamsAs1DForOutWhenUnconnected=off
  wires:
  Logical Operator/1 -> main_inj_on_off_signal/1  "main_inj_on_off_signal"
  Time_for_1_Degree/1 -> Divide/2
  Relational Operator/1 -> Logical Operator/1
  Main_Inj_trg_angle_inj2/1 -> Add/1
  Add/1 -> Relational Operator1/2  "Total_On_Degree"
  Cam_angle/1 -> Relational Operator1/1, Relational Operator/1
  Main_Inj_trg_angle_inj1/1 -> Relational Operator/2
  Relational Operator1/1 -> Logical Operator/2
  Total_ontime_maininjection/1 -> Divide/1
  Divide/1 -> Add/2

== system Project_Model_simulink_version_7_7_2023/CRDI_Integrated_Fuel_Injection_system/Injector_Subsystem/Injector1/Injector_2Subsystem/Pre_injection ==
  Cam_angle : Inport  OutDataTypeStr=single
  Total_ontime_preinjection : Inport  Port=2  OutDataTypeStr=single
  Time_For_1_Degree : Inport  Port=3  OutDataTypeStr=single
  Add : Sum  AccumDataTypeStr=single
      settings: AttributesFormatString=AccumDataTypeStr=%<AccumDataTypeStr>
  Divide : Product  Inputs=*/  OutDataTypeStr=single
  Logical Operator : Logic  AllPortsSameDT=off  OutDataTypeStr=boolean
  Pre_Inj_trg_angle_inj1 : Constant  Value=177.5
  Pre_Inj_trg_angle_inj2 : Constant  Value=177.5
  Relational Operator : RelationalOperator  OutDataTypeStr=boolean  RndMeth=Simplest
  Relational Operator1 : RelationalOperator  Operator=<=  OutDataTypeStr=boolean  RndMeth=Simplest
  pre_inj_on_off_signal : Outport  VectorParamsAs1DForOutWhenUnconnected=off
  wires:
  Divide/1 -> Add/2
  Relational Operator1/1 -> Logical Operator/2
  Pre_Inj_trg_angle_inj1/1 -> Relational Operator/2  "<Trigger_angle>"
  Total_ontime_preinjection/1 -> Divide/1
  Add/1 -> Relational Operator1/2  "Total_On_Degree"
  Pre_Inj_trg_angle_inj2/1 -> Add/1  "<Trigger_angle>"
  Time_For_1_Degree/1 -> Divide/2
  Relational Operator/1 -> Logical Operator/1
  Cam_angle/1 -> Relational Operator1/1, Relational Operator/1
  Logical Operator/1 -> pre_inj_on_off_signal/1  "pre_inj_on_off_signal"

== system Project_Model_simulink_version_7_7_2023/CRDI_Integrated_Fuel_Injection_system/Injector_Subsystem/Injector1/Injector_2Subsystem/Subsystem ==
  note: Subsystem
      | Description: Integrates Pre, Main, Post Injection to single output
      | Input: On time for pre Injection, On time for main Injection, On time for post Injection, Pre Pulse, Main Pulse, Post Pulse
      | Output: On time for Injection
  On_Time_Pre_Injection : Inport
  Pre_Pulse : Inport  Port=2
  On_Time_Main_Injection : Inport  Port=3
  Main_Pulse : Inport  Port=4
  Constant : Constant  Value=0  OutDataTypeStr=single
  Switch1 : Switch  Criteria=u2 ~= 0
  Switch2 : Switch  Criteria=u2 ~= 0
  Enable_Disable : Outport  OutDataTypeStr=single  VectorParamsAs1DForOutWhenUnconnected=off
  wires:
  Main_Pulse/1 -> Switch2/2
  On_Time_Main_Injection/1 -> Switch2/1
  Pre_Pulse/1 -> Switch1/2
  On_Time_Pre_Injection/1 -> Switch1/1
  Switch1/1 -> Enable_Disable/1  "On_Time_Injection"
  Constant/1 -> Switch2/3  "constant"
  Switch2/1 -> Switch1/3

== system Project_Model_simulink_version_7_7_2023/CRDI_Integrated_Fuel_Injection_system/Injector_Subsystem/Injector2/Injector_2Subsystem/If Action Subsystem ==
  In1 : Inport  OutDataTypeStr=single
  Action Port : ActionPort  ActionPortLabel=if(u1~=0)
  Out1 : Outport  OutDataTypeStr=single
  wires:
  In1/1 -> Out1/1

== system Project_Model_simulink_version_7_7_2023/CRDI_Integrated_Fuel_Injection_system/Injector_Subsystem/Injector2/Injector_2Subsystem/If Action Subsystem1 ==
  In1 : Inport  OutDataTypeStr=single
  Action Port : ActionPort  ActionPortLabel=elseif(u1==0)
  Out1 : Outport  OutDataTypeStr=single
  wires:
  In1/1 -> Out1/1

== system Project_Model_simulink_version_7_7_2023/CRDI_Integrated_Fuel_Injection_system/Injector_Subsystem/Injector2/Injector_2Subsystem/Main_injection ==
  Crank_angle : Inport  OutDataTypeStr=single
  Total_ontime_maininjection : Inport  Port=2  OutDataTypeStr=single
  Time_for_1_Degree : Inport  Port=3  OutDataTypeStr=single
  Add : Sum  AccumDataTypeStr=single
      settings: AttributesFormatString=AccumDataTypeStr=%<AccumDataTypeStr>
  Divide : Product  Inputs=*/  OutDataTypeStr=single
  Logical Operator : Logic  AllPortsSameDT=off  OutDataTypeStr=boolean
  Main_Inj_trg_angle_inj1 : Constant  Value=315
  Main_Inj_trg_angle_inj2 : Constant  Value=315
  Relational Operator : RelationalOperator  OutDataTypeStr=boolean  RndMeth=Simplest
  Relational Operator1 : RelationalOperator  Operator=<=  OutDataTypeStr=boolean  RndMeth=Simplest
  main_inj_on_off_signal : Outport  VectorParamsAs1DForOutWhenUnconnected=off
  wires:
  Logical Operator/1 -> main_inj_on_off_signal/1  "main_inj_on_off_signal"
  Time_for_1_Degree/1 -> Divide/2
  Relational Operator/1 -> Logical Operator/1
  Main_Inj_trg_angle_inj2/1 -> Add/1
  Add/1 -> Relational Operator1/2  "Total_On_Degree"
  Crank_angle/1 -> Relational Operator1/1, Relational Operator/1
  Main_Inj_trg_angle_inj1/1 -> Relational Operator/2
  Relational Operator1/1 -> Logical Operator/2
  Total_ontime_maininjection/1 -> Divide/1
  Divide/1 -> Add/2

== system Project_Model_simulink_version_7_7_2023/CRDI_Integrated_Fuel_Injection_system/Injector_Subsystem/Injector2/Injector_2Subsystem/Pre_injection ==
  Crank_angle : Inport  OutDataTypeStr=single
  Total_ontime_preinjection : Inport  Port=2  OutDataTypeStr=single
  Time_For_1_Degree : Inport  Port=3  OutDataTypeStr=single
  Add : Sum  AccumDataTypeStr=single
      settings: AttributesFormatString=AccumDataTypeStr=%<AccumDataTypeStr>
  Divide : Product  Inputs=*/  OutDataTypeStr=single
  Logical Operator : Logic  AllPortsSameDT=off  OutDataTypeStr=boolean
  Pre_Inj_trg_angle_inj1 : Constant  Value=312.5
  Pre_Inj_trg_angle_inj2 : Constant  Value=312.5
  Relational Operator : RelationalOperator  OutDataTypeStr=boolean  RndMeth=Simplest
  Relational Operator1 : RelationalOperator  Operator=<=  OutDataTypeStr=boolean  RndMeth=Simplest
  pre_inj_on_off_signal : Outport  VectorParamsAs1DForOutWhenUnconnected=off
  wires:
  Divide/1 -> Add/2
  Relational Operator1/1 -> Logical Operator/2
  Pre_Inj_trg_angle_inj1/1 -> Relational Operator/2  "<Trigger_angle>"
  Total_ontime_preinjection/1 -> Divide/1
  Add/1 -> Relational Operator1/2  "Total_On_Degree"
  Pre_Inj_trg_angle_inj2/1 -> Add/1  "<Trigger_angle>"
  Time_For_1_Degree/1 -> Divide/2
  Relational Operator/1 -> Logical Operator/1
  Crank_angle/1 -> Relational Operator1/1, Relational Operator/1
  Logical Operator/1 -> pre_inj_on_off_signal/1  "pre_inj_on_off_signal"

== system Project_Model_simulink_version_7_7_2023/CRDI_Integrated_Fuel_Injection_system/Injector_Subsystem/Injector2/Injector_2Subsystem/Subsystem ==
  note: Subsystem
      | Description: Integrates Pre, Main, Post Injection to single output
      | Input: On time for pre Injection, On time for main Injection, On time for post Injection, Pre Pulse, Main Pulse, Post Pulse
      | Output: On time for Injection
  On_Time_Pre_Injection : Inport
  Pre_Pulse : Inport  Port=2
  On_Time_Main_Injection : Inport  Port=3
  Main_Pulse : Inport  Port=4
  Constant : Constant  Value=0
  Switch1 : Switch  Criteria=u2 ~= 0
  Switch2 : Switch  Criteria=u2 ~= 0
  Enable_Disable : Outport  VectorParamsAs1DForOutWhenUnconnected=off
  wires:
  Main_Pulse/1 -> Switch2/2
  On_Time_Main_Injection/1 -> Switch2/1
  Pre_Pulse/1 -> Switch1/2
  On_Time_Pre_Injection/1 -> Switch1/1
  Switch1/1 -> Enable_Disable/1  "On_Time_Injection"
  Constant/1 -> Switch2/3  "constant"
  Switch2/1 -> Switch1/3

== system Project_Model_simulink_version_7_7_2023/CRDI_Integrated_Fuel_Injection_system/Injector_Subsystem/Injector3/Injector_2Subsystem/If Action Subsystem ==
  In1 : Inport  OutDataTypeStr=single
  Action Port : ActionPort  ActionPortLabel=if(u1~=0)
  Out1 : Outport  OutDataTypeStr=single
  wires:
  In1/1 -> Out1/1

== system Project_Model_simulink_version_7_7_2023/CRDI_Integrated_Fuel_Injection_system/Injector_Subsystem/Injector3/Injector_2Subsystem/If Action Subsystem1 ==
  In1 : Inport  OutDataTypeStr=single
  Action Port : ActionPort  ActionPortLabel=elseif(u1==0)
  Out1 : Outport  OutDataTypeStr=single
  wires:
  In1/1 -> Out1/1

== system Project_Model_simulink_version_7_7_2023/CRDI_Integrated_Fuel_Injection_system/Injector_Subsystem/Injector3/Injector_2Subsystem/Main_injection ==
  Crank_angle : Inport  OutDataTypeStr=single
  Total_ontime_maininjection : Inport  Port=2  OutDataTypeStr=single
  Time_for_1_Degree : Inport  Port=3  OutDataTypeStr=single
  Add : Sum  AccumDataTypeStr=single
      settings: AttributesFormatString=AccumDataTypeStr=%<AccumDataTypeStr>
  Divide : Product  Inputs=*/  OutDataTypeStr=single
  Logical Operator : Logic  AllPortsSameDT=off  OutDataTypeStr=boolean
  Main_Inj_trg_angle_inj1 : Constant  Value=225
  Main_Inj_trg_angle_inj2 : Constant  Value=225
  Relational Operator : RelationalOperator  OutDataTypeStr=boolean  RndMeth=Simplest
  Relational Operator1 : RelationalOperator  Operator=<=  OutDataTypeStr=boolean  RndMeth=Simplest
  main_inj_on_off_signal : Outport  VectorParamsAs1DForOutWhenUnconnected=off
  wires:
  Logical Operator/1 -> main_inj_on_off_signal/1  "main_inj_on_off_signal"
  Time_for_1_Degree/1 -> Divide/2
  Relational Operator/1 -> Logical Operator/1
  Main_Inj_trg_angle_inj2/1 -> Add/1
  Add/1 -> Relational Operator1/2  "Total_On_Degree"
  Crank_angle/1 -> Relational Operator1/1, Relational Operator/1
  Main_Inj_trg_angle_inj1/1 -> Relational Operator/2
  Relational Operator1/1 -> Logical Operator/2
  Total_ontime_maininjection/1 -> Divide/1
  Divide/1 -> Add/2

== system Project_Model_simulink_version_7_7_2023/CRDI_Integrated_Fuel_Injection_system/Injector_Subsystem/Injector3/Injector_2Subsystem/Pre_injection ==
  Crank_angle : Inport  OutDataTypeStr=single
  Total_ontime_preinjection : Inport  Port=2  OutDataTypeStr=single
  Time_For_1_Degree : Inport  Port=3  OutDataTypeStr=single
  Add : Sum  AccumDataTypeStr=single
      settings: AttributesFormatString=AccumDataTypeStr=%<AccumDataTypeStr>
  Divide : Product  Inputs=*/  OutDataTypeStr=single
  Logical Operator : Logic  AllPortsSameDT=off  OutDataTypeStr=boolean
  Pre_Inj_trg_angle_inj1 : Constant  Value=222.5
  Pre_Inj_trg_angle_inj2 : Constant  Value=222.5
  Relational Operator : RelationalOperator  OutDataTypeStr=boolean  RndMeth=Simplest
  Relational Operator1 : RelationalOperator  Operator=<=  OutDataTypeStr=boolean  RndMeth=Simplest
  pre_inj_on_off_signal : Outport  VectorParamsAs1DForOutWhenUnconnected=off
  wires:
  Divide/1 -> Add/2
  Relational Operator1/1 -> Logical Operator/2
  Pre_Inj_trg_angle_inj1/1 -> Relational Operator/2  "<Trigger_angle>"
  Total_ontime_preinjection/1 -> Divide/1
  Add/1 -> Relational Operator1/2  "Total_On_Degree"
  Pre_Inj_trg_angle_inj2/1 -> Add/1  "<Trigger_angle>"
  Time_For_1_Degree/1 -> Divide/2
  Relational Operator/1 -> Logical Operator/1
  Crank_angle/1 -> Relational Operator1/1, Relational Operator/1
  Logical Operator/1 -> pre_inj_on_off_signal/1  "pre_inj_on_off_signal"

== system Project_Model_simulink_version_7_7_2023/CRDI_Integrated_Fuel_Injection_system/Injector_Subsystem/Injector3/Injector_2Subsystem/Subsystem ==
  note: Subsystem
      | Description: Integrates Pre, Main, Post Injection to single output
      | Input: On time for pre Injection, On time for main Injection, On time for post Injection, Pre Pulse, Main Pulse, Post Pulse
      | Output: On time for Injection
  On_Time_Pre_Injection : Inport
  Pre_Pulse : Inport  Port=2
  On_Time_Main_Injection : Inport  Port=3
  Main_Pulse : Inport  Port=4
  Constant : Constant  Value=0
  Switch1 : Switch  Criteria=u2 ~= 0
  Switch2 : Switch  Criteria=u2 ~= 0
  Enable_Disable : Outport  VectorParamsAs1DForOutWhenUnconnected=off
  wires:
  Main_Pulse/1 -> Switch2/2
  On_Time_Main_Injection/1 -> Switch2/1
  Pre_Pulse/1 -> Switch1/2
  On_Time_Pre_Injection/1 -> Switch1/1
  Switch1/1 -> Enable_Disable/1  "On_Time_Injection"
  Constant/1 -> Switch2/3  "constant"
  Switch2/1 -> Switch1/3

== system Project_Model_simulink_version_7_7_2023/CRDI_Integrated_Fuel_Injection_system/Injector_Subsystem/Injector4/Injector_2Subsystem/If Action Subsystem ==
  In1 : Inport  OutDataTypeStr=single
  Action Port : ActionPort  ActionPortLabel=if(u1~=0)
  Out1 : Outport  OutDataTypeStr=single
  wires:
  In1/1 -> Out1/1

== system Project_Model_simulink_version_7_7_2023/CRDI_Integrated_Fuel_Injection_system/Injector_Subsystem/Injector4/Injector_2Subsystem/If Action Subsystem1 ==
  In1 : Inport  OutDataTypeStr=single
  Action Port : ActionPort  ActionPortLabel=elseif(u1==0)
  Out1 : Outport  OutDataTypeStr=single
  wires:
  In1/1 -> Out1/1

== system Project_Model_simulink_version_7_7_2023/CRDI_Integrated_Fuel_Injection_system/Injector_Subsystem/Injector4/Injector_2Subsystem/Main_injection ==
  Crank_angle : Inport  OutDataTypeStr=single
  Total_ontime_maininjection : Inport  Port=2  OutDataTypeStr=single
  Time_for_1_Degree : Inport  Port=3  OutDataTypeStr=single
  Add : Sum  AccumDataTypeStr=single
      settings: AttributesFormatString=AccumDataTypeStr=%<AccumDataTypeStr>
  Divide : Product  Inputs=*/  OutDataTypeStr=single
  Logical Operator : Logic  AllPortsSameDT=off  OutDataTypeStr=boolean
  Main_Inj_trg_angle_inj1 : Constant  Value=270
  Main_Inj_trg_angle_inj2 : Constant  Value=270
  Relational Operator : RelationalOperator  OutDataTypeStr=boolean  RndMeth=Simplest
  Relational Operator1 : RelationalOperator  Operator=<=  OutDataTypeStr=boolean  RndMeth=Simplest
  main_inj_on_off_signal : Outport  VectorParamsAs1DForOutWhenUnconnected=off
  wires:
  Logical Operator/1 -> main_inj_on_off_signal/1  "main_inj_on_off_signal"
  Time_for_1_Degree/1 -> Divide/2
  Relational Operator/1 -> Logical Operator/1
  Main_Inj_trg_angle_inj2/1 -> Add/1
  Add/1 -> Relational Operator1/2  "Total_On_Degree"
  Crank_angle/1 -> Relational Operator1/1, Relational Operator/1
  Main_Inj_trg_angle_inj1/1 -> Relational Operator/2
  Relational Operator1/1 -> Logical Operator/2
  Total_ontime_maininjection/1 -> Divide/1
  Divide/1 -> Add/2
